simulink model "Simscape_Benchmark_SIM1"  (R2021a)
settings: Solver=ode45  StartTime=0.0  StopTime=PHASE.Ttotal  FixedStep=Benchmark.Sim.Tint  RelTol=1e-5  AbsTol=1e-6
undefined symbols (not defined in the file): Actuators, Analysis, antisym, Benchmark, Bus, Disturbance, FSM, IntialCond, ISOL, K_Coarse_disc_t, Kslew_opt_disc_zoh, Model, MPS, PAYLOAD, PHASE, PMA, RWIsol, RWS, SA, Sensors, Slew, slosh, thr, X, Y, Z
libraries: sm_lib x215, nesl_utility x148, simulink x65, cstblocks x36, sharedtransform x4, vrlib x3, RCTblocks x1
(part 7 of 9)

== system Simscape_Benchmark_SIM1/Output to Workspace/FSM to Workspace ==
  Input : Inport
  Enable : EnablePort
  To Workspace42 : ToWorkspace  VariableName=cmd2FSM  SampleTime=Model.PayloadMeas_sampling.Ts
      settings: Save2DSignal=2-D array (concatenate along first dimension)
  wires:
  Input/1 -> To Workspace42/1

== system Simscape_Benchmark_SIM1/Output to Workspace/FSM to Workspace 1 ==
  Input : Inport
  Input1 : Inport  Port=2
  Enable : EnablePort
  To Workspace61 : ToWorkspace  VariableName=FSM_thetax  SampleTime=Model.PayloadMeas_sampling.Ts
      settings: Save2DSignal=2-D array (concatenate along first dimension)
  To Workspace62 : ToWorkspace  VariableName=FSM_thetay  SampleTime=Model.PayloadMeas_sampling.Ts
      settings: Save2DSignal=2-D array (concatenate along first dimension)
  wires:
  Input1/1 -> To Workspace62/1
  Input/1 -> To Workspace61/1

== system Simscape_Benchmark_SIM1/Output to Workspace/MPS to Workspace ==
  Input : Inport
  Enable : EnablePort
  To Workspace42 : ToWorkspace  VariableName=cmd2MPS  SampleTime=Model.PayloadMeas_sampling.Ts
      settings: Save2DSignal=2-D array (concatenate along first dimension)
  wires:
  Input/1 -> To Workspace42/1

== system Simscape_Benchmark_SIM1/Output to Workspace/Moving Average2 ==
  In1 : Inport
  Ground1 : Ground
  Terminator1 : Terminator
  Out1 : Outport
  wires:
  Ground1/1 -> Out1/1
  In1/1 -> Terminator1/1

== system Simscape_Benchmark_SIM1/Output to Workspace/Moving Average3 ==
  In1 : Inport
  Ground1 : Ground
  Terminator1 : Terminator
  Out1 : Outport
  wires:
  Ground1/1 -> Out1/1
  In1/1 -> Terminator1/1

== system Simscape_Benchmark_SIM1/Output to Workspace/Moving Average4 ==
  In1 : Inport
  Ground1 : Ground
  Terminator1 : Terminator
  Out1 : Outport
  wires:
  Ground1/1 -> Out1/1
  In1/1 -> Terminator1/1

== system Simscape_Benchmark_SIM1/Output to Workspace/Moving Average5 ==
  In1 : Inport
  Ground1 : Ground
  Terminator1 : Terminator
  Out1 : Outport
  wires:
  Ground1/1 -> Out1/1
  In1/1 -> Terminator1/1

== system Simscape_Benchmark_SIM1/Output to Workspace/Moving Average6 ==
  In1 : Inport
  Ground1 : Ground
  Terminator1 : Terminator
  Out1 : Outport
  wires:
  Ground1/1 -> Out1/1
  In1/1 -> Terminator1/1

== system Simscape_Benchmark_SIM1/Output to Workspace/Moving Average7 ==
  In1 : Inport
  Ground1 : Ground
  Terminator1 : Terminator
  Out1 : Outport
  wires:
  Ground1/1 -> Out1/1
  In1/1 -> Terminator1/1

== system Simscape_Benchmark_SIM1/Output to Workspace/OUTPUT RW DISTURBANCES DUE TO STATIC//DYNAMIC UNBALANCES ==
  In1 : Inport
  In2 : Inport  Port=2
  In3 : Inport  Port=3
  In4 : Inport  Port=4
  Enable : EnablePort
  To Workspace56 : ToWorkspace  VariableName=RW1_dist_at_revolute  SampleTime=Model.PayloadMeas_sampling.Ts
      settings: Save2DSignal=2-D array (concatenate along first dimension)
  To Workspace57 : ToWorkspace  VariableName=RW2_dist_at_revolute  SampleTime=Model.PayloadMeas_sampling.Ts
      settings: Save2DSignal=2-D array (concatenate along first dimension)
  To Workspace58 : ToWorkspace  VariableName=RW3_dist_at_revolute  SampleTime=Model.PayloadMeas_sampling.Ts
      settings: Save2DSignal=2-D array (concatenate along first dimension)
  To Workspace59 : ToWorkspace  VariableName=RW4_dist_at_revolute  SampleTime=Model.PayloadMeas_sampling.Ts
      settings: Save2DSignal=2-D array (concatenate along first dimension)
  wires:
  In1/1 -> To Workspace56/1
  In2/1 -> To Workspace57/1
  In4/1 -> To Workspace59/1
  In3/1 -> To Workspace58/1

== system Simscape_Benchmark_SIM1/Output to Workspace/PMA to Workspace ==
  In1 : Inport
  In2 : Inport  Port=2
  In3 : Inport  Port=3
  In4 : Inport  Port=4
  In5 : Inport  Port=5
  In6 : Inport  Port=6
  In7 : Inport  Port=7
  In8 : Inport  Port=8
  In9 : Inport  Port=9
  In10 : Inport  Port=10
  In11 : Inport  Port=11
  In12 : Inport  Port=12
  Enable : EnablePort
  To Workspace34 : ToWorkspace  VariableName=PMA_fz1  SampleTime=Model.PayloadMeas_sampling.Ts
      settings: Save2DSignal=2-D array (concatenate along first dimension)
  To Workspace35 : ToWorkspace  VariableName=PMA_fz2  SampleTime=Model.PayloadMeas_sampling.Ts
      settings: Save2DSignal=2-D array (concatenate along first dimension)
  To Workspace36 : ToWorkspace  VariableName=PMA_fz3  SampleTime=Model.PayloadMeas_sampling.Ts
      settings: Save2DSignal=2-D array (concatenate along first dimension)
  To Workspace37 : ToWorkspace  VariableName=PMA_fz4  SampleTime=Model.PayloadMeas_sampling.Ts
      settings: Save2DSignal=2-D array (concatenate along first dimension)
  To Workspace38 : ToWorkspace  VariableName=PMA_fz5  SampleTime=Model.PayloadMeas_sampling.Ts
      settings: Save2DSignal=2-D array (concatenate along first dimension)
  To Workspace39 : ToWorkspace  VariableName=PMA_fz6  SampleTime=Model.PayloadMeas_sampling.Ts
      settings: Save2DSignal=2-D array (concatenate along first dimension)
  To Workspace46 : ToWorkspace  VariableName=PMA_x1  SampleTime=Model.PayloadMeas_sampling.Ts
      settings: Save2DSignal=2-D array (concatenate along first dimension)
  To Workspace47 : ToWorkspace  VariableName=PMA_x2  SampleTime=Model.PayloadMeas_sampling.Ts
      settings: Save2DSignal=2-D array (concatenate along first dimension)
  To Workspace48 : ToWorkspace  VariableName=PMA_x3  SampleTime=Model.PayloadMeas_sampling.Ts
      settings: Save2DSignal=2-D array (concatenate along first dimension)
  To Workspace49 : ToWorkspace  VariableName=PMA_x4  SampleTime=Model.PayloadMeas_sampling.Ts
      settings: Save2DSignal=2-D array (concatenate along first dimension)
  To Workspace50 : ToWorkspace  VariableName=PMA_x5  SampleTime=Model.PayloadMeas_sampling.Ts
      settings: Save2DSignal=2-D array (concatenate along first dimension)
  To Workspace51 : ToWorkspace  VariableName=PMA_x6  SampleTime=Model.PayloadMeas_sampling.Ts
      settings: Save2DSignal=2-D array (concatenate along first dimension)
  wires:
  In2/1 -> To Workspace35/1
  In1/1 -> To Workspace34/1
  In9/1 -> To Workspace48/1
  In11/1 -> To Workspace50/1
  In8/1 -> To Workspace47/1
  In10/1 -> To Workspace49/1
  In3/1 -> To Workspace36/1
  In12/1 -> To Workspace51/1
  In5/1 -> To Workspace38/1
  In4/1 -> To Workspace37/1
  In6/1 -> To Workspace39/1
  In7/1 -> To Workspace46/1

== system Simscape_Benchmark_SIM1/Output to Workspace/PMA to Workspace 2 ==
  Input : Inport
  Enable : EnablePort
  To Workspace43 : ToWorkspace  VariableName=cmd2PMA  SampleTime=Model.PayloadMeas_sampling.Ts
      settings: Save2DSignal=2-D array (concatenate along first dimension)
  wires:
  Input/1 -> To Workspace43/1

== system Simscape_Benchmark_SIM1/Output to Workspace/RCS to Worskspace ==
  In1 : Inport
  In2 : Inport  Port=2
  In3 : Inport  Port=3
  Enable : EnablePort
  To Workspace12 : ToWorkspace  VariableName=RCS_OutAllocation  SampleTime=-1
      settings: Save2DSignal=2-D array (concatenate along first dimension)
  To Workspace70 : ToWorkspace  VariableName=RCS_active_Allocation  SampleTime=-1
      settings: Save2DSignal=2-D array (concatenate along first dimension)
  To Workspace77 : ToWorkspace  VariableName=RCS_cmd2Thrusters  SampleTime=-1
      settings: Save2DSignal=2-D array (concatenate along first dimension)
  wires:
  In3/1 -> To Workspace77/1
  In2/1 -> To Workspace12/1
  In1/1 -> To Workspace70/1

== system Simscape_Benchmark_SIM1/Sensors/Accelerometer Mirror 1 ==
  Xddot_M1 : Inport
  Rate Transition : RateTransition  OutPortSampleTime=Sensors.ACCm1.SampleTime
  Sensors.ACCm1.SelectSim : Gain  Gain=Sensors.ACCm1.SelectSim
  Sensors.ACCm1.highpass : cstblocks/LTI System  sys=Sensors.ACCm1.highpass  IC=[]
  Sensors.ACCm1.highpass1 : cstblocks/LTI System  sys=Sensors.ACCm1.highpass  IC=[]
  Sum : Sum  Inputs=|++
  acc_M1 : Subsystem
  Measurement : Outport
  Noise : Outport  Port=2
  wires:
  Sensors.ACCm1.SelectSim/1 -> Sum/2, Sensors.ACCm1.highpass1/1
  Xddot_M1/1 -> Rate Transition/1
  Sum/1 -> Sensors.ACCm1.highpass/1
  Sensors.ACCm1.highpass/1 -> Measurement/1  "with noise after filter"
  acc_M1/1(Out1) -> Sensors.ACCm1.SelectSim/1
  Sensors.ACCm1.highpass1/1 -> Noise/1
  Rate Transition/1 -> Sum/1  "after zoh"

== system Simscape_Benchmark_SIM1/Sensors/Accelerometer Mirror 2 ==
  Xddot_M2 : Inport
  Rate Transition1 : RateTransition  OutPortSampleTime=Sensors.ACCm2.SampleTime
  Sensors.ACCm2.SelectSim : Gain  Gain=Sensors.ACCm2.SelectSim
  Sensors.ACCm2.highpass1 : cstblocks/LTI System  sys=Sensors.ACCm2.highpass  IC=[]
  Sensors.ACCm2.highpass2 : cstblocks/LTI System  sys=Sensors.ACCm2.highpass  IC=[]
  Sum : Sum  Inputs=|++
  acc_M2 : Subsystem
  Measurement : Outport
  Noise : Outport  Port=2
  wires:
  Sum/1 -> Sensors.ACCm2.highpass1/1
  Sensors.ACCm2.SelectSim/1 -> Sensors.ACCm2.highpass2/1, Sum/2
  acc_M2/1(Out1) -> Sensors.ACCm2.SelectSim/1
  Sensors.ACCm2.highpass1/1 -> Measurement/1
  Xddot_M2/1 -> Rate Transition1/1
  Rate Transition1/1 -> Sum/1
  Sensors.ACCm2.highpass2/1 -> Noise/1

== system Simscape_Benchmark_SIM1/Sensors/Accelerometer at detector ==
  Xddot_detector : Inport
  Rate Transition1 : RateTransition  OutPortSampleTime=Sensors.ACCdect.SampleTime
  Sensors.ACCdect.SelectSim : Gain  Gain=Sensors.ACCdect.SelectSim
  Sensors.ACCdect.highpass : cstblocks/LTI System  sys=Sensors.ACCdect.highpass  IC=[]
  Sensors.ACCdect.highpass1 : cstblocks/LTI System  sys=Sensors.ACCdect.highpass  IC=[]
  Sum : Sum  Inputs=|++
  acc_dect : Subsystem
  Measurement : Outport
  Noise : Outport  Port=2
  wires:
  Sum/1 -> Sensors.ACCdect.highpass/1
  acc_dect/1(Out1) -> Sensors.ACCdect.SelectSim/1
  Rate Transition1/1 -> Sum/1
  Sensors.ACCdect.SelectSim/1 -> Sensors.ACCdect.highpass1/1, Sum/2
  Sensors.ACCdect.highpass/1 -> Measurement/1
  Xddot_detector/1 -> Rate Transition1/1
  Sensors.ACCdect.highpass1/1 -> Noise/1

== system Simscape_Benchmark_SIM1/Sensors/Fine Guidance Sensor (FGS) ==
  In1 : Inport
  FGS noise : Subsystem
  "Sensors.FGS.SelectSim " : Gain  Gain=Sensors.FGS.SelectSim
  Sum : Sum  Inputs=|++
  Zero-Order Hold : ZeroOrderHold  SampleTime=1/(Sensors.FGS.Bandwidth/(2*pi))
  Measurement : Outport
  Noise : Outport  Port=2
  wires:
  Sum/1 -> Measurement/1
  In1/1 -> Zero-Order Hold/1
  FGS noise/1(Out1) -> "Sensors.FGS.SelectSim "/1
  Zero-Order Hold/1 -> Sum/1
  "Sensors.FGS.SelectSim "/1 -> Noise/1, Sum/2

== system Simscape_Benchmark_SIM1/Sensors/Gyro (Coarse//fine) ==
  note: Note: gyro scale factor not included in the model
  In1 : Inport
  Noise - Corse gyro : Subsystem
  Noise Fine Gyro : Subsystem
  Rate Transition : RateTransition  OutPortSampleTime=Model.ACS_sampling.Ts
  Sensors.GYROc.SelectSim : Gain  Gain=Sensors.GYROc.SelectSim
  "Sensors.GYROf.SelectSim " : Gain  Gain=Sensors.GYROf.SelectSim
  Sum : Sum  Inputs=|++
  Sum1 : Sum  Inputs=|++
  Zero-Order Hold : ZeroOrderHold  SampleTime=1/(Sensors.GYROc.Bandwidth/(2*pi))
  Measurement : Outport
  Noise : Outport  Port=2
  wires:
  In1/1 -> Zero-Order Hold/1
  Sum/1 -> Rate Transition/1
  Sum1/1 -> Noise/1, Sum/2
  Zero-Order Hold/1 -> Sum/1
  Sensors.GYROc.SelectSim/1 -> Sum1/1
  "Sensors.GYROf.SelectSim "/1 -> Sum1/2
  Noise Fine Gyro/1(Out1) -> "Sensors.GYROf.SelectSim "/1
  Noise - Corse gyro/1(Out1) -> Sensors.GYROc.SelectSim/1
  Rate Transition/1 -> Measurement/1

== system Simscape_Benchmark_SIM1/Sensors/RW tachometer ==
  RW_omega : Inport
  RW speed measurement noise : Subsystem
  Rate Transition : RateTransition  OutPortSampleTime=0.05
  Sensors.RW_tachometer.SelectSim : Gain  Gain=Sensors.RW_tachometer.SelectSim
  Sum : Sum  Inputs=|++
  Out1 : Outport
  wires:
  Sum/1 -> Out1/1
  RW_omega/1 -> Rate Transition/1
  Rate Transition/1 -> Sum/1
  RW speed measurement noise/1(Out1) -> Sensors.RW_tachometer.SelectSim/1
  Sensors.RW_tachometer.SelectSim/1 -> Sum/2

== system Simscape_Benchmark_SIM1/Sensors/Rotation measurements of the fast steering mirror (FSM) ==
  THETAxy : Inport
  FGS noise : Subsystem
  Rate Transition4 : RateTransition  OutPortSampleTime=Model.PayloadMeas_sampling.Ts
  "Sensors.FGS.SelectSim " : Gain  Gain=Sensors.FGS.SelectSim
  Sum : Sum  Inputs=|++
  Measurement : Outport
  Noise : Outport  Port=2
  wires:
  THETAxy/1 -> Rate Transition4/1
  FGS noise/1(Out1) -> "Sensors.FGS.SelectSim "/1
  "Sensors.FGS.SelectSim "/1 -> Sum/2, Noise/1
  Rate Transition4/1 -> Sum/1
  Sum/1 -> Measurement/1

== system Simscape_Benchmark_SIM1/Sensors/Star tracker ==
  Eul_Angles : Inport
  Rate Transition : RateTransition  OutPortSampleTime=Model.ACS_sampling.Ts
  SST noise : Subsystem
  "Sensors.SST.SelectSim " : Gain  Gain=Sensors.SST.SelectSim
  Sum : Sum  Inputs=|++
  Measurement : Outport
  Noise : Outport  Port=2
  wires:
  Sum/1 -> Measurement/1
  Rate Transition/1 -> Sum/1
  "Sensors.SST.SelectSim "/1 -> Noise/1, Sum/2
  Eul_Angles/1 -> Rate Transition/1
  SST noise/1(Out1) -> "Sensors.SST.SelectSim "/1

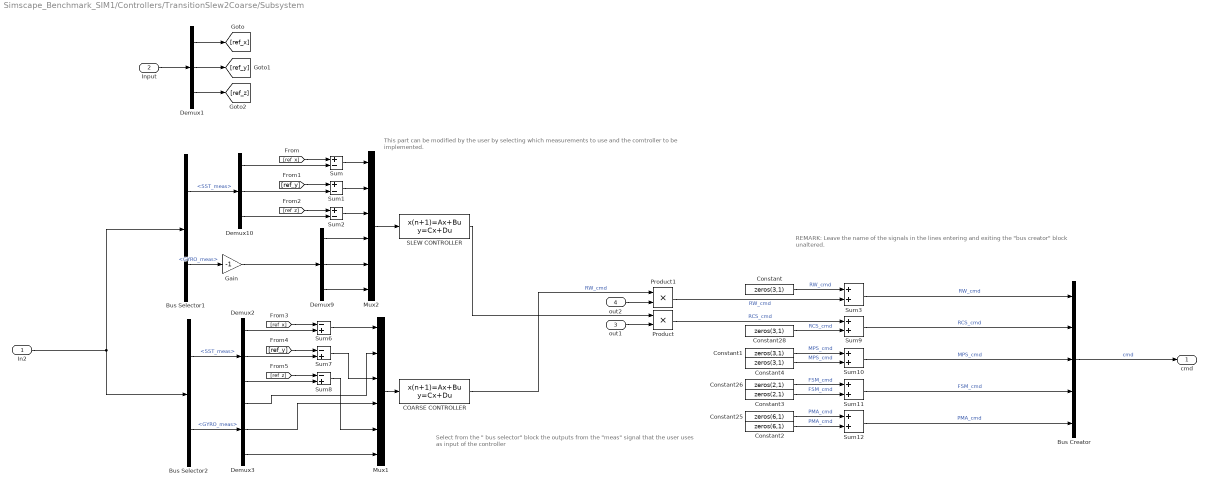
== system Simscape_Benchmark_SIM1/Controllers/TransitionSlew2Coarse/Subsystem ==
  note: This part can be modified by the user by selecting which measurements to use and the comtroller to be implemented.
  note: REMARK: Leave the name of the signals in the lines entering and exiting the "bus creator" block unaltered.
  note: Select from the " bus selector" block the outputs from the "meas" signal that the user uses as input of the controller
  In2 : Inport
  Input : Inport  Port=2
  out1 : Inport  Port=3
  out2 : Inport  Port=4
  Bus Creator : BusCreator  Inputs=5
  Bus Selector1 : BusSelector  OutputSignals=SST_meas,GYRO_meas
  Bus Selector2 : BusSelector  OutputSignals=SST_meas,GYRO_meas
  COARSE CONTROLLER : DiscreteStateSpace  A=K_Coarse_disc_t.A  B=K_Coarse_disc_t.B  C=K_Coarse_disc_t.C  D=K_Coarse_disc_t.D  SampleTime=Model.ACS_sampling.Ts
  Constant : Constant  Value=zeros(3,1)  SampleTime=Model.ACS_sampling.Ts
  Constant1 : Constant  Value=zeros(3,1)  SampleTime=Model.MPS_sampling.Ts
  Constant2 : Constant  Value=zeros(6,1)  SampleTime=Model.PayloadMeas_sampling.Ts
  Constant25 : Constant  Value=zeros(6,1)  SampleTime=Model.PayloadMeas_sampling.Ts
  Constant26 : Constant  Value=zeros(2,1)  SampleTime=Model.PayloadMeas_sampling.Ts
  Constant28 : Constant  Value=zeros(3,1)  SampleTime=Model.ACS_sampling.Ts
  Constant3 : Constant  Value=zeros(2,1)  SampleTime=Model.PayloadMeas_sampling.Ts
  Constant4 : Constant  Value=zeros(3,1)  SampleTime=Model.MPS_sampling.Ts
  Demux{1..3,9..10} (5 alike) : Demux  Outputs=3
  Gain : Gain  Gain=-1
  Mux1 : Mux  Inputs=6
  Mux2 : Mux  Inputs=6
  Product : Product
  Product1 : Product
  SLEW CONTROLLER : DiscreteStateSpace  A=Kslew_opt_disc_zoh.A  B=Kslew_opt_disc_zoh.B  C=Kslew_opt_disc_zoh.C  D=Kslew_opt_disc_zoh.D  SampleTime=Model.ACS_sampling.Ts
  Sum : Sum  Inputs=+-
  Sum1 : Sum  Inputs=+-
  Sum{3,9..12} (5 alike) : Sum
  Sum2 : Sum  Inputs=+-
  Sum6 : Sum  Inputs=-+
  Sum7 : Sum  Inputs=-+
  Sum8 : Sum  Inputs=-+
  cmd : Outport
  wires:
  Demux10/2 -> Sum1/2
  Bus Selector1/1 -> Demux10/1  "<SST_meas>"
  [ref_z] -> Sum8/1
  Constant4/1 -> Sum10/2  "MPS_cmd"
  Gain/1 -> Demux9/1
  Demux9/1 -> Mux2/4
  Sum/1 -> Mux2/1
  Demux3/2 -> Mux1/4
  Mux2/1 -> SLEW CONTROLLER/1
  Sum8/1 -> Mux1/5
  SLEW CONTROLLER/1 -> Product/1
  Constant26/1 -> Sum11/1  "FSM_cmd"
  Demux10/3 -> Sum2/2
  Constant1/1 -> Sum10/1  "MPS_cmd"
  Sum2/1 -> Mux2/3
  Sum12/1 -> Bus Creator/5  "PMA_cmd"
  Sum1/1 -> Mux2/2
  Mux1/1 -> COARSE CONTROLLER/1
  Bus Selector1/2 -> Gain/1  "<GYRO_meas>"
  Constant25/1 -> Sum12/1  "PMA_cmd"
  [ref_x] -> Sum/1
  Demux9/3 -> Mux2/6
  Constant2/1 -> Sum12/2  "PMA_cmd"
  Demux3/1 -> Mux1/2
  Demux9/2 -> Mux2/5
  Demux2/2 -> Sum7/2
  [ref_z] -> Sum2/1
  Constant/1 -> Sum3/1  "RW_cmd"
  Constant28/1 -> Sum9/2  "RCS_cmd"
  Demux2/3 -> Sum8/2
  Product/1 -> Sum9/1  "RCS_cmd"
  Bus Creator/1 -> cmd/1  "cmd"
  Constant3/1 -> Sum11/2  "FSM_cmd"
  Sum3/1 -> Bus Creator/1  "RW_cmd"
  Sum10/1 -> Bus Creator/3  "MPS_cmd"
  Sum7/1 -> Mux1/3
  Sum9/1 -> Bus Creator/2  "RCS_cmd"
  Sum11/1 -> Bus Creator/4  "FSM_cmd"
  [ref_y] -> Sum1/1
  [ref_x] -> Sum6/1
  In2/1 -> Bus Selector2/1, Bus Selector1/1
  Bus Selector2/2 -> Demux3/1  "<GYRO_meas>"
  out2/1 -> Product1/2
  [ref_y] -> Sum7/1
  Demux10/1 -> Sum/2
  Demux2/1 -> Sum6/2
  Bus Selector2/1 -> Demux2/1  "<SST_meas>"
  Demux3/3 -> Mux1/6
  Product1/1 -> Sum3/2  "RW_cmd"
  Demux1/3 -> [ref_z]
  Demux1/1 -> [ref_x]
  Demux1/2 -> [ref_y]
  Input/1 -> Demux1/1
  out1/1 -> Product/2
  Sum6/1 -> Mux1/1
  COARSE CONTROLLER/1 -> Product1/1  "RW_cmd"

== system Simscape_Benchmark_SIM1/Dynamical system/MPS model/MPS (thruster model) ==
  Cmd_force : Inport  PortDimensions=3
  Cmd_Torque : Inport  Port=2  PortDimensions=3
  2nd order system : cstblocks/LTI System  sys=tf(Actuators.MPS.om^2,[1 2*Actuators.MPS.damp*Actuators.MPS.om (Actuators.MPS.om)^2])*eye(MPS.nb_thr)  IC=[]
  Allocation Function (Updated) : MATLABFcn  MATLABFcn=MPS_AllocationFunct  OutputDimensions=MPS.nb_thr+1
  Constant10 : Constant  Value=MPS.sc_thrust_Ht_reshaped'
  Constant11 : Constant  Value=MPS.nb_thr
  Constant13 : Constant  Value=MPS.F
  Constant9 : Constant  Value=MPS.sc_thrust_Hf_reshaped'
  Demux1 : Demux  Outputs=[thr.nb_thr,1]
  Gain : Gain  Gain=MPS.F
  Mux : Mux  Inputs=2
  Mux2 : Mux  Inputs=2
  Mux3 : Mux  Inputs=[6,1,1,thr.nb_thr*3,thr.nb_thr*3]
  Quantizer1 : Quantizer  QuantizationInterval=MPS.res
  Saturation1 : Saturate  UpperLimit=MPS.F  LowerLimit=-MPS.F
  Terminator : Terminator
  Thr_ForceMPS : Outport
  wires:
  Constant10/1 -> Mux3/5  "thr.nb_thr*3"
  Constant9/1 -> Mux3/4  "thr.nb_thr*3"
  Mux2/1 -> Mux3/1
  Constant13/1 -> Mux3/3  "1"
  Demux1/1 -> Gain/1  "U_cont"
  Mux3/1 -> Mux/1
  Allocation Function (Updated)/1 -> Demux1/1
  Constant11/1 -> Mux3/2  "1"
  Cmd_force/1 -> Mux2/1
  Cmd_Torque/1 -> Mux2/2
  Mux/1 -> Allocation Function (Updated)/1
  Demux1/2 -> Terminator/1  "n_activated"
  Saturation1/1 -> Quantizer1/1
  Quantizer1/1 -> 2nd order system/1
  2nd order system/1 -> Thr_ForceMPS/1
  Gain/1 -> Saturation1/1, Mux/2

== system Simscape_Benchmark_SIM1/Dynamical system/Payload System (Telescope structure, FSM, PMA system, Isolator)/Fast-Steering Mirror ==
  theta_x_cmd : Inport
  theta_y_cmd : Inport  Port=2
  FSM plate : sm_lib/Body Elements/Brick Solid  GraphicAmbientColor=[0.15 0.15 0.15 1.0]  BasedOnType=Density  BrickDimensions=[0.08 0.08 0.005]  BrickDimensionUnits=m  CenterOfMass=[0 0 0]  CenterOfMassUnits=m  GraphicDiffuseColor=[1.0 1.0 0.0]  Density=1000  DensityUnits=kg/m^3  DoExposeReferenceFrame=on  GraphicEmissiveColor=[0.0 0.0 0.0 1.0]  ExportEntireGeometry=off  SerializedFrames=<Frames/>  MarkerShape=Sphere  MarkerSize=10  GraphicType=FromGeometry  InertiaType=Custom  Mass=FSM.m  MassUnits=kg  MomentsOfInertia=diag(FSM.IatG)  MomentsOfInertiaUnits=kg*m^2  GraphicOpacity=1.0  ProductsOfInertia=[0 0 0]  ProductsOfInertiaUnits=kg*m^2  GraphicShininess=75  GraphicSpecularColor=[0.5 0.5 0.5 1.0]  GraphicVisPropType=SimpleVisualProperties
  Gain4 : Gain  Gain=FSM.k
  Gain5 : Gain  Gain=FSM.d
  Gain6 : Gain  Gain=FSM.k
  Gain7 : Gain  Gain=FSM.d
  Mux5 : Mux  Inputs=2
  Mux6 : Mux  Inputs=2
  Mux7 : Mux  Inputs=2
  PS-Simulink Converter{24..29} (6 alike) : nesl_utility/PS-Simulink Converter  PhysicalDomain=network_engine_domain  SubClassName=ps_output  LeftPortType=input  RightPortType=output  PseudoPeriodic=off  Frequencies=[]  Unit=inherit  AffineConversion=off
      settings: SourceProductBaseCode=PW,SS
  Simulink-PS Converter8 : nesl_utility/Simulink-PS Converter  PhysicalDomain=network_engine_domain  SubClassName=ps_input  LeftPortType=input  RightPortType=output  PseudoPeriodic=off  Frequencies=[]  NoiseDistribution=none  NoiseParameters=[]  Unit=1  AffineConversion=off  FilteringAndDerivatives=provide  SimscapeFilterOrder=2  InputFilterTimeConstant=0.001  UdotUserProvided=0
      settings: SourceProductBaseCode=PW,SS
  Simulink-PS Converter9 : nesl_utility/Simulink-PS Converter  PhysicalDomain=network_engine_domain  SubClassName=ps_input  LeftPortType=input  RightPortType=output  PseudoPeriodic=off  Frequencies=[]  NoiseDistribution=none  NoiseParameters=[]  Unit=1  AffineConversion=off  FilteringAndDerivatives=provide  SimscapeFilterOrder=2  InputFilterTimeConstant=0.001  UdotUserProvided=0
      settings: SourceProductBaseCode=PW,SS
  Sum{4..7} (4 alike) : Sum  Inputs=|+-
  Universal Joint FSM : sm_lib/Joints/Universal Joint  JointMode=Normal  SenseConstraintForce=off  SenseConstraintForceX=off  SenseConstraintForceY=off  SenseConstraintForceZ=off  SenseConstraintTorque=off  SenseConstraintTorqueX=off  SenseConstraintTorqueY=off  SenseConstraintTorqueZ=off  SenseTotalForce=off  SenseTotalForceX=off  SenseTotalForceY=off  SenseTotalForceZ=off  SenseTotalTorque=off  SenseTotalTorqueX=off  SenseTotalTorqueY=off  SenseTotalTorqueZ=off  CompositeWrenchDir=FollowerOnBase  CompositeWrenchFrame=BaseFrame  RxEquilibriumPosition=0  RxEquilibriumPositionUnits=rad  RxSpringStiffness=0  RxSpringStiffnessUnits=N*m/rad  RxDampingCoefficient=0  RxDampingCoefficientUnits=N*m/(rad/s)  RxTorqueActuationMode=InputTorque  RxMotionActuationMode=ComputedMotion  RxSensePosition=on  RxSenseVelocity=on  RxSenseAcceleration=on  RxSenseTorqueForce=off  RxSenseLowerLimitTorqueForce=off  RxSenseUpperLimitTorqueForce=off  RxLowerLimitSpecify=off  RxLowerLimitBound=-Actuators.FSM.MaxRotation  RxLowerLimitBoundUnits=rad  RxLowerLimitStiffness=1e4  RxLowerLimitStiffnessUnits=N*m/deg  RxLowerLimitDamping=10  RxLowerLimitDampingUnits=N*m/(deg/s)  RxLowerLimitTransitionRegionWidth=0.1  RxLowerLimitTransitionRegionWidthUnits=deg  RxUpperLimitSpecify=off  RxUpperLimitBound=Actuators.FSM.MaxRotation  RxUpperLimitBoundUnits=rad  RxUpperLimitStiffness=1e4  RxUpperLimitStiffnessUnits=N*m/deg  RxUpperLimitDamping=10  RxUpperLimitDampingUnits=N*m/(deg/s)  RxUpperLimitTransitionRegionWidth=0.1  RxUpperLimitTransitionRegionWidthUnits=deg  RxPositionTargetSpecify=on  RxPositionTargetPriority=High  RxPositionTargetValue=0  RxPositionTargetValueUnits=deg  RxVelocityTargetSpecify=on  RxVelocityTargetPriority=High  RxVelocityTargetValue=0  RxVelocityTargetValueUnits=deg/s  RyEquilibriumPosition=0  RyEquilibriumPositionUnits=deg  RySpringStiffness=0  RySpringStiffnessUnits=N*m/rad  RyDampingCoefficient=0  RyDampingCoefficientUnits=N*m/(rad/s)  RyTorqueActuationMode=InputTorque  RyMotionActuationMode=ComputedMotion  RySensePosition=on  RySenseVelocity=on  RySenseAcceleration=on  RySenseTorqueForce=off  RySenseLowerLimitTorqueForce=off  RySenseUpperLimitTorqueForce=off  RyLowerLimitSpecify=off  RyLowerLimitBound=-90  RyLowerLimitBoundUnits=deg  RyLowerLimitStiffness=1e4  RyLowerLimitStiffnessUnits=N*m/deg  RyLowerLimitDamping=10  RyLowerLimitDampingUnits=N*m/(deg/s)  RyLowerLimitTransitionRegionWidth=0.1  RyLowerLimitTransitionRegionWidthUnits=deg  RyUpperLimitSpecify=off  RyUpperLimitBound=90  RyUpperLimitBoundUnits=deg  RyUpperLimitStiffness=1e4  RyUpperLimitStiffnessUnits=N*m/deg  RyUpperLimitDamping=10  RyUpperLimitDampingUnits=N*m/(deg/s)  RyUpperLimitTransitionRegionWidth=0.1  RyUpperLimitTransitionRegionWidthUnits=deg  RyPositionTargetSpecify=on  RyPositionTargetPriority=High  RyPositionTargetValue=0  RyPositionTargetValueUnits=deg  RyVelocityTargetSpecify=on  RyVelocityTargetPriority=High  RyVelocityTargetValue=0  RyVelocityTargetValueUnits=deg/s
  Universal Joint FSM2 : sm_lib/Joints/Universal Joint  Commented=on  JointMode=Normal  SenseConstraintForce=off  SenseConstraintForceX=off  SenseConstraintForceY=off  SenseConstraintForceZ=off  SenseConstraintTorque=off  SenseConstraintTorqueX=off  SenseConstraintTorqueY=off  SenseConstraintTorqueZ=off  SenseTotalForce=off  SenseTotalForceX=off  SenseTotalForceY=off  SenseTotalForceZ=off  SenseTotalTorque=off  SenseTotalTorqueX=off  SenseTotalTorqueY=off  SenseTotalTorqueZ=off  CompositeWrenchDir=FollowerOnBase  CompositeWrenchFrame=BaseFrame  RxEquilibriumPosition=0  RxEquilibriumPositionUnits=rad  RxSpringStiffness=0  RxSpringStiffnessUnits=N*m/rad  RxDampingCoefficient=0  RxDampingCoefficientUnits=N*m/(rad/s)  RxTorqueActuationMode=InputTorque  RxMotionActuationMode=ComputedMotion  RxSensePosition=on  RxSenseVelocity=on  RxSenseAcceleration=on  RxSenseTorqueForce=off  RxSenseLowerLimitTorqueForce=off  RxSenseUpperLimitTorqueForce=off  RxLowerLimitSpecify=on  RxLowerLimitBound=-Actuators.FSM.MaxRotation  RxLowerLimitBoundUnits=rad  RxLowerLimitStiffness=1e4  RxLowerLimitStiffnessUnits=N*m/deg  RxLowerLimitDamping=10  RxLowerLimitDampingUnits=N*m/(deg/s)  RxLowerLimitTransitionRegionWidth=0.1  RxLowerLimitTransitionRegionWidthUnits=deg  RxUpperLimitSpecify=on  RxUpperLimitBound=Actuators.FSM.MaxRotation  RxUpperLimitBoundUnits=rad  RxUpperLimitStiffness=1e4  RxUpperLimitStiffnessUnits=N*m/deg  RxUpperLimitDamping=10  RxUpperLimitDampingUnits=N*m/(deg/s)  RxUpperLimitTransitionRegionWidth=0.1  RxUpperLimitTransitionRegionWidthUnits=deg  RxPositionTargetSpecify=on  RxPositionTargetPriority=High  RxPositionTargetValue=0  RxPositionTargetValueUnits=deg  RxVelocityTargetSpecify=on  RxVelocityTargetPriority=High  RxVelocityTargetValue=0  RxVelocityTargetValueUnits=deg/s  RyEquilibriumPosition=0  RyEquilibriumPositionUnits=deg  RySpringStiffness=0  RySpringStiffnessUnits=N*m/rad  RyDampingCoefficient=0  RyDampingCoefficientUnits=N*m/(rad/s)  RyTorqueActuationMode=InputTorque  RyMotionActuationMode=ComputedMotion  RySensePosition=on  RySenseVelocity=on  RySenseAcceleration=on  RySenseTorqueForce=off  RySenseLowerLimitTorqueForce=off  RySenseUpperLimitTorqueForce=off  RyLowerLimitSpecify=off  RyLowerLimitBound=-90  RyLowerLimitBoundUnits=deg  RyLowerLimitStiffness=1e4  RyLowerLimitStiffnessUnits=N*m/deg  RyLowerLimitDamping=10  RyLowerLimitDampingUnits=N*m/(deg/s)  RyLowerLimitTransitionRegionWidth=0.1  RyLowerLimitTransitionRegionWidthUnits=deg  RyUpperLimitSpecify=off  RyUpperLimitBound=90  RyUpperLimitBoundUnits=deg  RyUpperLimitStiffness=1e4  RyUpperLimitStiffnessUnits=N*m/deg  RyUpperLimitDamping=10  RyUpperLimitDampingUnits=N*m/(deg/s)  RyUpperLimitTransitionRegionWidth=0.1  RyUpperLimitTransitionRegionWidthUnits=deg  RyPositionTargetSpecify=on  RyPositionTargetPriority=High  RyPositionTargetValue=0  RyPositionTargetValueUnits=deg  RyVelocityTargetSpecify=on  RyVelocityTargetPriority=High  RyVelocityTargetValue=0  RyVelocityTargetValueUnits=deg/s
  Universal Joint FSM1 : PMIOPort  Side=Left
  ang_acc : Outport
  ang_vel : Outport  Port=2
  rot : Outport  Port=3
  theta_X : Outport  Port=4
  theta_Y : Outport  Port=5
  wires:
  Mux5/1 -> ang_acc/1
  PS-Simulink Converter29/1 -> Mux5/2
  PS-Simulink Converter26/1 -> Mux5/1
  Sum7/1 -> Simulink-PS Converter9/1
  PS-Simulink Converter25/1 -> Mux6/1, Gain5/1
  PS-Simulink Converter27/1 -> Sum5/2, theta_Y/1, Mux7/2
  theta_x_cmd/1 -> Sum4/1
  PS-Simulink Converter24/1 -> theta_X/1, Mux7/1, Sum4/2
  Sum6/1 -> Simulink-PS Converter8/1
  PS-Simulink Converter28/1 -> Gain7/1, Mux6/2
  Gain7/1 -> Sum7/2
  Gain6/1 -> Sum7/1
  Sum4/1 -> Gain4/1
  Sum5/1 -> Gain6/1
  Gain4/1 -> Sum6/1
  Gain5/1 -> Sum6/2
  Mux7/1 -> rot/1
  theta_y_cmd/1 -> Sum5/1
  Mux6/1 -> ang_vel/1
  connections:
  FSM plate/RConn1 -- Universal Joint FSM/RConn1
  PS-Simulink Converter25/LConn1 -- Universal Joint FSM/RConn3
  Universal Joint FSM/RConn5 -- PS-Simulink Converter27/LConn1
  Universal Joint FSM/RConn4 -- PS-Simulink Converter26/LConn1
  Universal Joint FSM/RConn6 -- PS-Simulink Converter28/LConn1
  Simulink-PS Converter8/RConn1 -- Universal Joint FSM/LConn2
  Universal Joint FSM/RConn7 -- PS-Simulink Converter29/LConn1
  PS-Simulink Converter24/LConn1 -- Universal Joint FSM/RConn2
  Simulink-PS Converter9/RConn1 -- Universal Joint FSM/LConn3
  Universal Joint FSM1/RConn1 -- Universal Joint FSM/LConn1

== system Simscape_Benchmark_SIM1/Dynamical system/Payload System (Telescope structure, FSM, PMA system, Isolator)/Integration ==
  In1 : Inport
  Constant2 : Constant  Value=IntialCond.Q0
  Demux11 : Demux  Outputs=[3,3]
  Integrator2 : Integrator
  Mux19 : Mux  Inputs=2
  Quaternion Integration2 : Subsystem
  Quaternions to Rotation Angles2 : sharedtransform/Quaternions to Rotation Angles  rotationOrder=XYZ  aMode=aMode
      settings: SourceProductBaseCode=AE,PW,DR,MT,UV,VE
  Out1 : Outport
  wires:
  Demux11/1 -> Mux19/1
  Demux11/2 -> Quaternion Integration2/1(om)
  Constant2/1 -> Quaternion Integration2/2(Q_init)
  Integrator2/1 -> Demux11/1
  Quaternions to Rotation Angles2/1 -> Mux19/2
  Quaternion Integration2/1(q_4) -> Quaternions to Rotation Angles2/1
  In1/1 -> Integrator2/1
  Mux19/1 -> Out1/1

== system Simscape_Benchmark_SIM1/Dynamical system/Payload System (Telescope structure, FSM, PMA system, Isolator)/Integration 1 ==
  In1 : Inport
  Constant1 : Constant  Value=IntialCond.Q0
  Demux9 : Demux  Outputs=[3,3]
  Integrator3 : Integrator
  Mux : Mux  Inputs=2
  Quaternion Integration1 : Subsystem
  Quaternions to Rotation Angles1 : sharedtransform/Quaternions to Rotation Angles  rotationOrder=XYZ  aMode=aMode
      settings: SourceProductBaseCode=AE,PW,DR,MT,UV,VE
  Out1 : Outport
  wires:
  Integrator3/1 -> Demux9/1
  Demux9/2 -> Quaternion Integration1/1(om)
  In1/1 -> Integrator3/1
  Constant1/1 -> Quaternion Integration1/2(Q_init)
  Quaternion Integration1/1(q_4) -> Quaternions to Rotation Angles1/1
  Quaternions to Rotation Angles1/1 -> Mux/2
  Demux9/1 -> Mux/1
  Mux/1 -> Out1/1

== system Simscape_Benchmark_SIM1/Dynamical system/Payload System (Telescope structure, FSM, PMA system, Isolator)/Optical sensitivity (FSM) ==
  inFSM : Inport
  Constant1 : Constant  Value=0
  Demux2 : Demux  Outputs=2
  Gain : Gain
  Gain1 : Gain
  Mux1 : Mux  Inputs=3
  Sensitivity matrix : Gain  Gain=PAYLOAD.Sensitivity_FSM([1,3],1:2)  Multiplication=Matrix(K*u) (u vector)
  Out1 : Outport
  wires:
  inFSM/1 -> Sensitivity matrix/1
  Constant1/1 -> Mux1/3
  Demux2/1 -> Gain1/1
  Sensitivity matrix/1 -> Demux2/1
  Mux1/1 -> Out1/1
  Demux2/2 -> Gain/1
  Gain/1 -> Mux1/1
  Gain1/1 -> Mux1/2

== system Simscape_Benchmark_SIM1/Dynamical system/Payload System (Telescope structure, FSM, PMA system, Isolator)/Optical sensitivity (M1 and M2) ==
  note: They are variation dr with respect to the nominal reflected ray from the FSM which has direction  [0 1 0] (note dr_y is zero);
      |
      | The demux-mux below transform the variation with respect to the initial LOS direction [0 0 1]
      |
      | ------   drx_reflected = dr_x= dtheta_y (across boresight)
      |
      | ------   drz_reflected = dr_y= dtheta_x (across boresight)
      |
      | ------   No additional contribution from the sensitivityies is given along y. (or  z - LOS direction- as expected); the sensitivities have all zero values in the second row.
  xdd_MPC : Inport
  Xddot,C1 : Inport  Port=2
  Xddot,C2 : Inport  Port=3
  xdd_MPC_Inertial : Inport  Port=4
  Constant : Constant  Value=0
  Constant1 : Constant  Value=0
  Demux : Demux  Outputs=[3,3]
  Demux1 : Demux  Outputs=3
  Demux2 : Demux  Outputs=3
  Demux3 : Demux  Outputs=[3,3]
  Demux4 : Demux  Outputs=[3,3]
  Gain : Gain
  Gain1 : Gain
  Mux : Mux  Inputs=3
  Mux1 : Mux  Inputs=3
  Mux2 : Mux  Inputs=2
  Mux3 : Mux  Inputs=2
  S1 : Gain  Gain=PAYLOAD.Sensitivity_M1  Multiplication=Matrix(K*u) (u vector)
  S2 : Gain  Gain=PAYLOAD.Sensitivity_M2  Multiplication=Matrix(K*u) (u vector)
  Sum : Sum  Inputs=+++
  Sum1 : Sum  Inputs=|+-
  Sum2 : Sum  Inputs=|+-
  Terminator : Terminator
  Terminator1 : Terminator
  Terminator2 : Terminator
  tau_02M1 : Gain  Gain=[eye(3), antisym([0.;0.;-0.2385]);zeros(3,3),eye(3)]  Multiplication=Matrix(K*u) (u vector)
  tau_02M2 : Gain  Gain=[eye(3), antisym([0;0;-1.126045]);zeros(3,3),eye(3)]  Multiplication=Matrix(K*u) (u vector)
  los_dd : Outport
  wires:
  Xddot,C1/1 -> Sum1/1  "M1"
  Sum/1 -> los_dd/1
  S1/1 -> Demux1/1
  Demux/1 -> Terminator/1
  Demux/2 -> Sum/3
  Demux1/1 -> Mux/2
  Demux1/3 -> Mux/1
  Mux/1 -> Gain1/1
  Mux1/1 -> Gain/1
  S2/1 -> Demux2/1
  Demux2/3 -> Mux1/1
  Demux2/1 -> Mux1/2
  Demux1/2 -> Terminator1/1
  Constant/1 -> Mux/3
  Constant1/1 -> Mux1/3
  Demux2/2 -> Terminator2/1
  Mux2/1 -> S1/1
  Demux3/1 -> Mux2/2
  Demux3/2 -> Mux2/1
  Demux4/2 -> Mux3/1
  Demux4/1 -> Mux3/2
  Mux3/1 -> S2/1
  Sum1/1 -> Demux3/1
  Sum2/1 -> Demux4/1
  tau_02M2/1 -> Sum2/2
  xdd_MPC/1 -> tau_02M2/1, tau_02M1/1
  Gain/1 -> Sum/2
  Gain1/1 -> Sum/1
  tau_02M1/1 -> Sum1/2
  Xddot,C2/1 -> Sum2/1
  xdd_MPC_Inertial/1 -> Demux/1

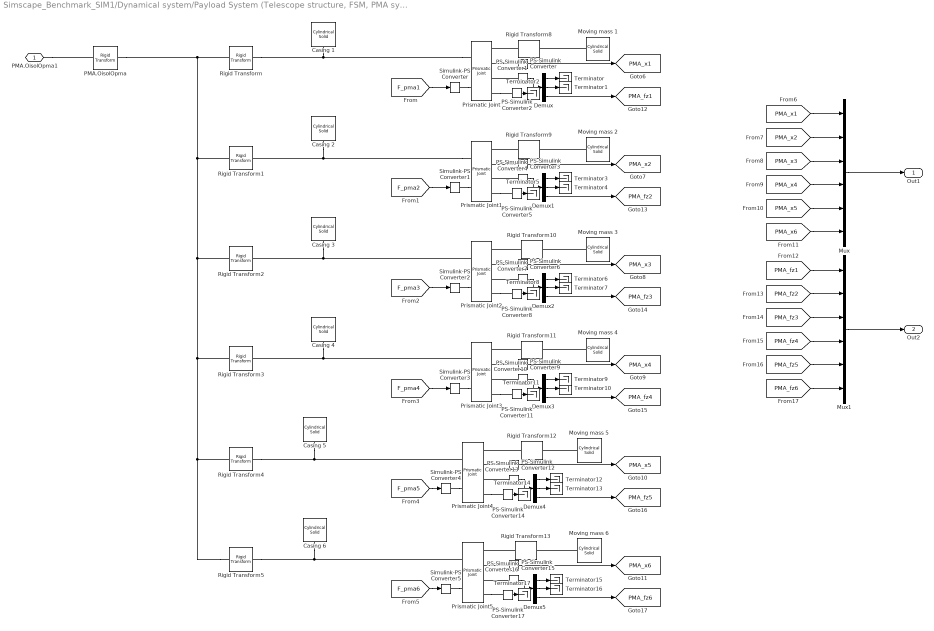
== system Simscape_Benchmark_SIM1/Dynamical system/Payload System (Telescope structure, FSM, PMA system, Isolator)/Proof-Mass Actuator system ==
  Casing {1..6} (6 alike) : sm_lib/Body Elements/Cylindrical Solid  GraphicAmbientColor=[0.15 0.15 0.15 1.0]  BasedOnType=Density  CenterOfMass=PMA.Sim.OsimGcasing  CenterOfMassUnits=m  GraphicDiffuseColor=[0.5 0.5 0.5]  CylinderLength=PMA.l  CylinderLengthUnits=m  CylinderRadius=PMA.Sim.Rcasing  CylinderRadiusUnits=m  Density=1000  DensityUnits=kg/m^3  DoExposeReferenceFrame=off  GraphicEmissiveColor=[0.0 0.0 0.0 1.0]  ExportEntireGeometry=off  SerializedFrames=<Frames><Frame><Id>Frame1</Id><Value><Name>F1</Name><Origin><Source>GeometricFeature</Source><FeatureName>bottom surface</FeatureName></Origin><PrimaryAxis><DefinedDirection>+Z</DefinedDirection><Source>ReferenceFrame</Source><SourceDirection>+Z</SourceDirection><FeatureName></FeatureName></PrimaryAxis><SecondaryAxis><DefinedDirection>+X</DefinedDirection><Source>ReferenceFrame</Source><SourceDirection>+X</SourceDirection><FeatureName></FeatureName></SecondaryAxis></Value></Frame></Frames>  MarkerShape=Sphere  MarkerSize=10  GraphicType=FromGeometry  InertiaType=Custom  Mass=PMA.M-PMA.m  MassUnits=kg  MomentsOfInertia=diag(PMA.Sim.Icasing_Osim)  MomentsOfInertiaUnits=kg*m^2  GraphicOpacity=0.4  ProductsOfInertia=[PMA.Sim.Icasing_Osim(2,3);PMA.Sim.Icasing_Osim(3,1);PMA.Sim.Icasing_Osim(1,2)]  ProductsOfInertiaUnits=kg*m^2  GraphicShininess=75  GraphicSpecularColor=[0.5 0.5 0.5 1.0]  GraphicVisPropType=SimpleVisualProperties
  Demux{,1..5} (6 alike) : Demux  Outputs=3
  Moving mass {1..6} (6 alike) : sm_lib/Body Elements/Cylindrical Solid  GraphicAmbientColor=[0.15 0.15 0.15 1.0]  BasedOnType=Density  CenterOfMass=[0 0 0]  CenterOfMassUnits=m  GraphicDiffuseColor=[1.0 0.0 0.2]  CylinderLength=PMA.l*0.1  CylinderLengthUnits=m  CylinderRadius=PMA.Sim.Rcasing-PMA.Sim.Rcasing*0.2  CylinderRadiusUnits=m  Density=1000  DensityUnits=kg/m^3  DoExposeReferenceFrame=on  GraphicEmissiveColor=[0.0 0.0 0.0 1.0]  ExportEntireGeometry=off  SerializedFrames=<Frames/>  MarkerShape=Sphere  MarkerSize=10  GraphicType=FromGeometry  InertiaType=PointMass  Mass=PMA.m  MassUnits=kg  MomentsOfInertia=[1 1 1]  MomentsOfInertiaUnits=kg*m^2  GraphicOpacity=1  ProductsOfInertia=[0 0 0]  ProductsOfInertiaUnits=kg*m^2  GraphicShininess=75  GraphicSpecularColor=[0.5 0.5 0.5 1.0]  GraphicVisPropType=SimpleVisualProperties
  Mux : Mux  Inputs=6
  Mux1 : Mux  Inputs=6
  PMA.OisolOpma : sm_lib/Frames and Transforms/Rigid Transform  TranslationMethod=Cartesian  TranslationStandardOffset=0  TranslationLengthUnit=m  TranslationStandardAxis=+Z  TranslationCartesianOffset=PMA.OisolOpma  TranslationROffset=0  TranslationROffsetUnits=m  TranslationZOffset=0  TranslationZOffsetUnits=m  TranslationThetaOffset=0  TranslationThetaOffsetUnits=deg  RotationMethod=None  RotationAngleUnits=deg  RotationStandardAxis=+Z  RotationAngle=0.0  RotationArbitraryAxis=[0 0 1]  FollAlignAxisA=+X  BaseAlignAxisA=+Y  FollAlignAxisB=+Y  BaseAlignAxisB=+Z  RotationSequenceAxes=FollowerAxes  RotationSequence=XYX  RotationSequenceAngles=[0 0 0]  RotationSequenceAnglesUnits=deg  RotationMatrix=[1 0 0; 0 1 0; 0 0 1]
  PS-Simulink Converter{,1..17} (18 alike) : nesl_utility/PS-Simulink Converter  PhysicalDomain=network_engine_domain  SubClassName=ps_output  LeftPortType=input  RightPortType=output  PseudoPeriodic=off  Frequencies=[]  Unit=inherit  AffineConversion=off
      settings: SourceProductBaseCode=PW,SS
  Prismatic Joint{,1..5} (6 alike) : sm_lib/Joints/Prismatic Joint  JointMode=Normal  SenseConstraintForce=off  SenseConstraintForceX=off  SenseConstraintForceY=off  SenseConstraintForceZ=off  SenseConstraintTorque=off  SenseConstraintTorqueX=off  SenseConstraintTorqueY=off  SenseConstraintTorqueZ=off  SenseTotalForce=on  SenseTotalForceX=off  SenseTotalForceY=off  SenseTotalForceZ=off  SenseTotalTorque=on  SenseTotalTorqueX=off  SenseTotalTorqueY=off  SenseTotalTorqueZ=off  CompositeWrenchDir=FollowerOnBase  CompositeWrenchFrame=BaseFrame  EquilibriumPosition=0  EquilibriumPositionUnits=m  SpringStiffness=PMA.k  SpringStiffnessUnits=N/m  DampingCoefficient=PMA.d  DampingCoefficientUnits=N/(m/s)  TorqueActuationMode=InputTorque  MotionActuationMode=ComputedMotion  SensePosition=on  SenseVelocity=off  SenseAcceleration=off  SenseTorqueForce=off  SenseLowerLimitTorqueForce=off  SenseUpperLimitTorqueForce=off  LowerLimitSpecify=off  LowerLimitBound=-1  LowerLimitBoundUnits=m  LowerLimitStiffness=1e6  LowerLimitStiffnessUnits=N/m  LowerLimitDamping=1e3  LowerLimitDampingUnits=N/(m/s)  LowerLimitTransitionRegionWidth=1e-4  LowerLimitTransitionRegionWidthUnits=m  UpperLimitSpecify=off  UpperLimitBound=1  UpperLimitBoundUnits=m  UpperLimitStiffness=1e6  UpperLimitStiffnessUnits=N/m  UpperLimitDamping=1e3  UpperLimitDampingUnits=N/(m/s)  UpperLimitTransitionRegionWidth=1e-4  UpperLimitTransitionRegionWidthUnits=m  PositionTargetSpecify=on  PositionTargetPriority=High  PositionTargetValue=0  PositionTargetValueUnits=m  VelocityTargetSpecify=on  VelocityTargetPriority=High  VelocityTargetValue=0  VelocityTargetValueUnits=m/s
  Rigid Transform : sm_lib/Frames and Transforms/Rigid Transform  TranslationMethod=Cartesian  TranslationStandardOffset=0  TranslationLengthUnit=m  TranslationStandardAxis=+Z  TranslationCartesianOffset=PMA.pos1  TranslationROffset=0  TranslationROffsetUnits=m  TranslationZOffset=0  TranslationZOffsetUnits=m  TranslationThetaOffset=0  TranslationThetaOffsetUnits=deg  RotationMethod=None  RotationAngleUnits=deg  RotationStandardAxis=+Z  RotationAngle=0.0  RotationArbitraryAxis=[0 0 1]  FollAlignAxisA=+X  BaseAlignAxisA=+Y  FollAlignAxisB=+Y  BaseAlignAxisB=+Z  RotationSequenceAxes=FollowerAxes  RotationSequence=XYX  RotationSequenceAngles=[0 0 0]  RotationSequenceAnglesUnits=deg  RotationMatrix=[1 0 0; 0 1 0; 0 0 1]
  Rigid Transform1 : sm_lib/Frames and Transforms/Rigid Transform  TranslationMethod=Cartesian  TranslationStandardOffset=0  TranslationLengthUnit=m  TranslationStandardAxis=+Z  TranslationCartesianOffset=PMA.pos2  TranslationROffset=0  TranslationROffsetUnits=m  TranslationZOffset=0  TranslationZOffsetUnits=m  TranslationThetaOffset=0  TranslationThetaOffsetUnits=deg  RotationMethod=None  RotationAngleUnits=deg  RotationStandardAxis=+Z  RotationAngle=0.0  RotationArbitraryAxis=[0 0 1]  FollAlignAxisA=+X  BaseAlignAxisA=+Y  FollAlignAxisB=+Y  BaseAlignAxisB=+Z  RotationSequenceAxes=FollowerAxes  RotationSequence=XYX  RotationSequenceAngles=[0 0 0]  RotationSequenceAnglesUnits=deg  RotationMatrix=[1 0 0; 0 1 0; 0 0 1]
  Rigid Transform{8..13} (6 alike) : sm_lib/Frames and Transforms/Rigid Transform  TranslationMethod=Cartesian  TranslationStandardOffset=0  TranslationLengthUnit=m  TranslationStandardAxis=+Z  TranslationCartesianOffset=[0;0;PMA.Sim.O_CoM_moving(3)]  TranslationROffset=0  TranslationROffsetUnits=m  TranslationZOffset=0  TranslationZOffsetUnits=m  TranslationThetaOffset=0  TranslationThetaOffsetUnits=deg  RotationMethod=None  RotationAngleUnits=deg  RotationStandardAxis=+Z  RotationAngle=0.0  RotationArbitraryAxis=[0 0 1]  FollAlignAxisA=+X  BaseAlignAxisA=+Y  FollAlignAxisB=+Y  BaseAlignAxisB=+Z  RotationSequenceAxes=FollowerAxes  RotationSequence=XYX  RotationSequenceAngles=[0 0 0]  RotationSequenceAnglesUnits=deg  RotationMatrix=[1 0 0; 0 1 0; 0 0 1]
  Rigid Transform2 : sm_lib/Frames and Transforms/Rigid Transform  TranslationMethod=Cartesian  TranslationStandardOffset=0  TranslationLengthUnit=m  TranslationStandardAxis=+Z  TranslationCartesianOffset=PMA.pos3  TranslationROffset=0  TranslationROffsetUnits=m  TranslationZOffset=0  TranslationZOffsetUnits=m  TranslationThetaOffset=0  TranslationThetaOffsetUnits=deg  RotationMethod=None  RotationAngleUnits=deg  RotationStandardAxis=+Z  RotationAngle=0.0  RotationArbitraryAxis=[0 0 1]  FollAlignAxisA=+X  BaseAlignAxisA=+Y  FollAlignAxisB=+Y  BaseAlignAxisB=+Z  RotationSequenceAxes=FollowerAxes  RotationSequence=XYX  RotationSequenceAngles=[0 0 0]  RotationSequenceAnglesUnits=deg  RotationMatrix=[1 0 0; 0 1 0; 0 0 1]
  Rigid Transform3 : sm_lib/Frames and Transforms/Rigid Transform  TranslationMethod=Cartesian  TranslationStandardOffset=0  TranslationLengthUnit=m  TranslationStandardAxis=+Z  TranslationCartesianOffset=PMA.pos4  TranslationROffset=0  TranslationROffsetUnits=m  TranslationZOffset=0  TranslationZOffsetUnits=m  TranslationThetaOffset=0  TranslationThetaOffsetUnits=deg  RotationMethod=RotationMatrix  RotationAngleUnits=deg  RotationStandardAxis=+Z  RotationAngle=0.0  RotationArbitraryAxis=[0 0 1]  FollAlignAxisA=+X  BaseAlignAxisA=+Y  FollAlignAxisB=+Y  BaseAlignAxisB=+Z  RotationSequenceAxes=FollowerAxes  RotationSequence=XYX  RotationSequenceAngles=[0 0 0]  RotationSequenceAnglesUnits=deg  RotationMatrix=[1 0 0; 0 0 1; 0 -1 0]
  Rigid Transform4 : sm_lib/Frames and Transforms/Rigid Transform  TranslationMethod=Cartesian  TranslationStandardOffset=0  TranslationLengthUnit=m  TranslationStandardAxis=+Z  TranslationCartesianOffset=PMA.pos5  TranslationROffset=0  TranslationROffsetUnits=m  TranslationZOffset=0  TranslationZOffsetUnits=m  TranslationThetaOffset=0  TranslationThetaOffsetUnits=deg  RotationMethod=RotationMatrix  RotationAngleUnits=deg  RotationStandardAxis=+Z  RotationAngle=0.0  RotationArbitraryAxis=[0 0 1]  FollAlignAxisA=+X  BaseAlignAxisA=+Y  FollAlignAxisB=+Y  BaseAlignAxisB=+Z  RotationSequenceAxes=FollowerAxes  RotationSequence=XYX  RotationSequenceAngles=[0 0 0]  RotationSequenceAnglesUnits=deg  RotationMatrix=([1 0 0; 0 0 1; 0 -1 0]*[cosd(120) 0 -sind(120); 0 1 0; sind(120) 0 cosd(120)])
  Rigid Transform5 : sm_lib/Frames and Transforms/Rigid Transform  TranslationMethod=Cartesian  TranslationStandardOffset=0  TranslationLengthUnit=m  TranslationStandardAxis=+Z  TranslationCartesianOffset=PMA.pos6  TranslationROffset=0  TranslationROffsetUnits=m  TranslationZOffset=0  TranslationZOffsetUnits=m  TranslationThetaOffset=0  TranslationThetaOffsetUnits=deg  RotationMethod=RotationMatrix  RotationAngleUnits=deg  RotationStandardAxis=+Z  RotationAngle=0.0  RotationArbitraryAxis=[0 0 1]  FollAlignAxisA=+X  BaseAlignAxisA=+Y  FollAlignAxisB=+Y  BaseAlignAxisB=+Z  RotationSequenceAxes=FollowerAxes  RotationSequence=XYX  RotationSequenceAngles=[0 0 0]  RotationSequenceAnglesUnits=deg  RotationMatrix=([1 0 0; 0 0 1; 0 -1 0]*[cosd(240) 0 -sind(240); 0 1 0; sind(240) 0 cosd(240)])
  Simulink-PS Converter{,1..5} (6 alike) : nesl_utility/Simulink-PS Converter  PhysicalDomain=network_engine_domain  SubClassName=ps_input  LeftPortType=input  RightPortType=output  PseudoPeriodic=off  Frequencies=[]  NoiseDistribution=none  NoiseParameters=[]  Unit=1  AffineConversion=off  FilteringAndDerivatives=provide  SimscapeFilterOrder=1  InputFilterTimeConstant=0.001  UdotUserProvided=0
      settings: SourceProductBaseCode=PW,SS
  Terminator{,1..17} (18 alike) : Terminator
  PMA.OisolOpma1 : PMIOPort  Side=Left
  Out1 : Outport
  Out2 : Outport  Port=2
  tag scope: PMA_fz1=global, PMA_fz2=global, PMA_fz3=global, PMA_fz4=global, PMA_fz5=global, PMA_fz6=global, PMA_x1=global, PMA_x2=global, PMA_x3=global, PMA_x4=global, PMA_x5=global, PMA_x6=global
  wires:
  PS-Simulink Converter16/1 -> Demux5/1
  PS-Simulink Converter7/1 -> Demux2/1
  [PMA_fz3] -> Mux1/3
  [PMA_fz5] -> Mux1/5
  Demux/1 -> Terminator/1
  PS-Simulink Converter15/1 -> [PMA_x6]
  Demux2/3 -> [PMA_fz3]
  [F_pma3] -> Simulink-PS Converter2/1
  Demux4/2 -> Terminator13/1
  PS-Simulink Converter10/1 -> Demux3/1
  Demux1/1 -> Terminator3/1
  [PMA_x2] -> Mux/2
  Demux2/2 -> Terminator7/1
  PS-Simulink Converter13/1 -> Demux4/1
  Demux3/3 -> [PMA_fz4]
  [PMA_x4] -> Mux/4
  Demux2/1 -> Terminator6/1
  Demux4/1 -> Terminator12/1
  Demux3/1 -> Terminator9/1
  Demux/3 -> [PMA_fz1]
  [PMA_fz4] -> Mux1/4
  [F_pma2] -> Simulink-PS Converter1/1
  Demux5/2 -> Terminator16/1
  PS-Simulink Converter9/1 -> [PMA_x4]
  [PMA_fz6] -> Mux1/6
  PS-Simulink Converter3/1 -> [PMA_x2]
  [PMA_fz2] -> Mux1/2
  [PMA_x1] -> Mux/1
  PS-Simulink Converter/1 -> [PMA_x1]
  PS-Simulink Converter14/1 -> Terminator14/1
  Demux1/2 -> Terminator4/1
  PS-Simulink Converter5/1 -> Terminator5/1
  Demux4/3 -> [PMA_fz5]
  [F_pma4] -> Simulink-PS Converter3/1
  [F_pma5] -> Simulink-PS Converter4/1
  PS-Simulink Converter6/1 -> [PMA_x3]
  PS-Simulink Converter4/1 -> Demux1/1
  [PMA_x6] -> Mux/6
  Demux/2 -> Terminator1/1
  [PMA_x3] -> Mux/3
  Demux5/3 -> [PMA_fz6]
  Demux3/2 -> Terminator10/1
  PS-Simulink Converter12/1 -> [PMA_x5]
  [PMA_x5] -> Mux/5
  [PMA_fz1] -> Mux1/1
  Demux1/3 -> [PMA_fz2]
  [F_pma1] -> Simulink-PS Converter/1
  PS-Simulink Converter1/1 -> Demux/1
  PS-Simulink Converter11/1 -> Terminator11/1
  PS-Simulink Converter2/1 -> Terminator2/1
  [F_pma6] -> Simulink-PS Converter5/1
  PS-Simulink Converter8/1 -> Terminator8/1
  Demux5/1 -> Terminator15/1
  PS-Simulink Converter17/1 -> Terminator17/1
  Mux/1 -> Out1/1
  Mux1/1 -> Out2/1
  connections:
  Prismatic Joint3/RConn4 -- PS-Simulink Converter11/LConn1
  PS-Simulink Converter9/LConn1 -- Prismatic Joint3/RConn2
  Rigid Transform11/LConn1 -- Prismatic Joint3/RConn1
  Prismatic Joint/RConn4 -- PS-Simulink Converter2/LConn1
  Rigid Transform8/LConn1 -- Prismatic Joint/RConn1
  Rigid Transform9/LConn1 -- Prismatic Joint1/RConn1
  PS-Simulink Converter7/LConn1 -- Prismatic Joint2/RConn3
  Moving mass 3/RConn1 -- Rigid Transform10/RConn1
  Simulink-PS Converter3/RConn1 -- Prismatic Joint3/LConn2
  PS-Simulink Converter/LConn1 -- Prismatic Joint/RConn2
  Moving mass 1/RConn1 -- Rigid Transform8/RConn1
  Simulink-PS Converter/RConn1 -- Prismatic Joint/LConn2
  Rigid Transform10/LConn1 -- Prismatic Joint2/RConn1
  Simulink-PS Converter4/RConn1 -- Prismatic Joint4/LConn2
  Simulink-PS Converter5/RConn1 -- Prismatic Joint5/LConn2
  PS-Simulink Converter1/LConn1 -- Prismatic Joint/RConn3
  PS-Simulink Converter6/LConn1 -- Prismatic Joint2/RConn2
  Prismatic Joint1/LConn1 -- Casing 2/LConn1 -- Rigid Transform1/RConn1
  Prismatic Joint1/RConn4 -- PS-Simulink Converter5/LConn1
  Rigid Transform2/RConn1 -- Prismatic Joint2/LConn1 -- Casing 3/LConn1
  PS-Simulink Converter10/LConn1 -- Prismatic Joint3/RConn3
  Moving mass 5/RConn1 -- Rigid Transform12/RConn1
  PS-Simulink Converter3/LConn1 -- Prismatic Joint1/RConn2
  PS-Simulink Converter16/LConn1 -- Prismatic Joint5/RConn3
  PS-Simulink Converter4/LConn1 -- Prismatic Joint1/RConn3
  Rigid Transform3/RConn1 -- Prismatic Joint3/LConn1 -- Casing 4/LConn1
  Simulink-PS Converter2/RConn1 -- Prismatic Joint2/LConn2
  Rigid Transform13/LConn1 -- Prismatic Joint5/RConn1
  Rigid Transform4/RConn1 -- Prismatic Joint4/LConn1 -- Casing 5/LConn1
  Simulink-PS Converter1/RConn1 -- Prismatic Joint1/LConn2
  Prismatic Joint2/RConn4 -- PS-Simulink Converter8/LConn1
  PS-Simulink Converter12/LConn1 -- Prismatic Joint4/RConn2
  Rigid Transform5/LConn1 -- Rigid Transform/LConn1 -- PMA.OisolOpma/RConn1 -- Rigid Transform1/LConn1 -- Rigid Transform2/LConn1 -- Rigid Transform3/LConn1 -- Rigid Transform4/LConn1
  Moving mass 2/RConn1 -- Rigid Transform9/RConn1
  Prismatic Joint4/RConn4 -- PS-Simulink Converter14/LConn1
  PS-Simulink Converter15/LConn1 -- Prismatic Joint5/RConn2
  PS-Simulink Converter13/LConn1 -- Prismatic Joint4/RConn3
  Moving mass 6/RConn1 -- Rigid Transform13/RConn1
  Rigid Transform5/RConn1 -- Prismatic Joint5/LConn1 -- Casing 6/LConn1
  Moving mass 4/RConn1 -- Rigid Transform11/RConn1
  Prismatic Joint5/RConn4 -- PS-Simulink Converter17/LConn1
  Rigid Transform12/LConn1 -- Prismatic Joint4/RConn1
  Prismatic Joint/LConn1 -- Casing 1/LConn1 -- Rigid Transform/RConn1
  PMA.OisolOpma1/RConn1 -- PMA.OisolOpma/LConn1

== system Simscape_Benchmark_SIM1/Dynamical system/Payload System (Telescope structure, FSM, PMA system, Isolator)/Quaternion Integration ==
  om : Inport
  Q_init : Inport  Port=2
  Integrator6 : Integrator  InitialConditionSource=external
  Subsystem : Subsystem
  q_4 : Outport
  wires:
  Subsystem/1(Out1) -> Integrator6/1
  om/1 -> Subsystem/2(om)
  Integrator6/1 -> q_4/1, Subsystem/1(q_4)
  Q_init/1 -> Integrator6/2
